simulink library "robot"  (Simulink 7.4)
settings: Solver=ode45  StartTime=0.0  StopTime=10.0  RelTol=1e-3
libraries: AtomicLibrary x3, BusImpl x1
settings Model: Creator=andrey  LastModifiedBy=andrey

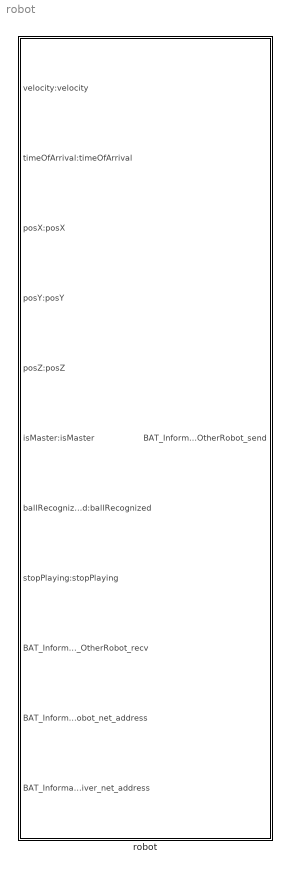
== system robot ==
  robot : Subsystem  Tag=id=_2CVEwKbHEeKVjd_905naCg

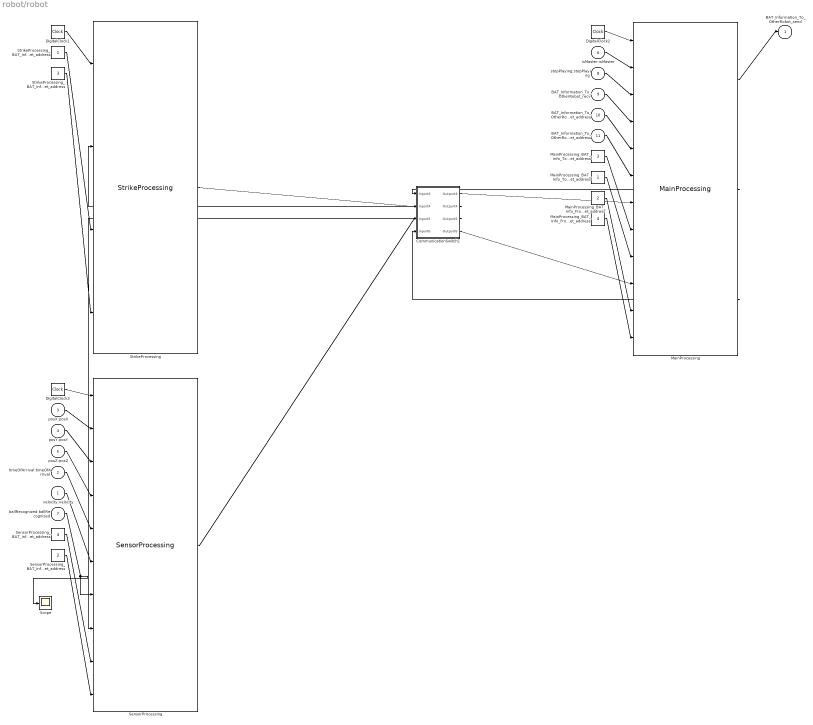
== system robot/robot ==
  velocity:velocity : Inport  Tag=id=_3IT1YKbHEeKVjd_905naCg  DataType=double  OutDataType=fixdt(1, 16)  OutScaling=2^0  OutDataTypeStr=double
  timeOfArrival:timeOfArrival : Inport  Tag=id=_3IliMKbHEeKVjd_905naCg  Port=2  DataType=double  OutDataType=fixdt(1, 16)  OutScaling=2^0  OutDataTypeStr=double
  posX:posX : Inport  Tag=id=_3I8HgKbHEeKVjd_905naCg  Port=3  DataType=double  OutDataType=fixdt(1, 16)  OutScaling=2^0  OutDataTypeStr=double
  posY:posY : Inport  Tag=id=_3JgvQKbHEeKVjd_905naCg  Port=4  DataType=double  OutDataType=fixdt(1, 16)  OutScaling=2^0  OutDataTypeStr=double
  posZ:posZ : Inport  Tag=id=_3KMEsKbHEeKVjd_905naCg  Port=5  DataType=double  OutDataType=fixdt(1, 16)  OutScaling=2^0  OutDataTypeStr=double
  isMaster:isMaster : Inport  Tag=id=_3Kp-wKbHEeKVjd_905naCg  Port=6  DataType=boolean  OutDataType=fixdt(1, 16)  OutScaling=2^0  OutDataTypeStr=boolean
  ballRecognized:ballRecognized : Inport  Tag=id=_3LJG8KbHEeKVjd_905naCg  Port=7  DataType=boolean  OutDataType=fixdt(1, 16)  OutScaling=2^0  OutDataTypeStr=boolean
  stopPlaying:stopPlaying : Inport  Tag=id=_3LnBAKbHEeKVjd_905naCg  Port=8  DataType=boolean  OutDataType=fixdt(1, 16)  OutScaling=2^0  OutDataTypeStr=boolean
  BAT_Information_To_OtherRobot_recv : Inport  Tag=id=_3MnGkKbHEeKVjd_905naCg  Port=9  UseBusObject=on  OutDataType=fixdt(1, 16)  OutScaling=2^0
      settings: BusObject=PacketBus
  BAT_Information_To_OtherRobot_net_address : Inport  Tag=id=_3MoUsKbHEeKVjd_905naCg  Port=10  DataType=uint8  OutDataType=fixdt(1, 16)  OutScaling=2^0  OutDataTypeStr=uint8
  BAT_Information_To_OtherRobot_receiver_net_address : Inport  Tag=id=_3MoUsabHEeKVjd_905naCg  Port=11  DataType=uint8  OutDataType=fixdt(1, 16)  OutScaling=2^0  OutDataTypeStr=uint8
  CommunicationSwitch1 : Subsystem  Tag=id=_2CVr0KbHEeKVjd_905naCg  LoadFcn=MainBusGenerator
  DigitalClock1 : DigitalClock  Tag=id=_2EqnEKbHEeKVjd_905naCg  SampleTime=0.0010
  DigitalClock2 : DigitalClock  Tag=id=_2ExUwKbHEeKVjd_905naCg  SampleTime=0.0010
  DigitalClock3 : DigitalClock  Tag=id=_2E1mMKbHEeKVjd_905naCg  SampleTime=0.0010
  MainProcessing : AtomicLibrary/MainProcessing  Tag=id=_2EwtsKbHEeKVjd_905naCg  SystemSampleTime=-1
  MainProcessing_BAT_Info_From_SensorProcessing1_net_address : Constant  Tag=id=_3Dm7kKbHEeKVjd_905naCg  Value=2  OutDataTypeMode=uint8  OutDataTypeStr=uint8
  MainProcessing_BAT_Info_From_SensorProcessing1_receiver_net_address : Constant  Tag=id=_4yrFcabHEeKVjd_905naCg  Value=4  OutDataTypeMode=uint8  OutDataTypeStr=uint8
  MainProcessing_BAT_Info_ToStrikeProcessing1_net_address : Constant  Tag=id=_3DVOwKbHEeKVjd_905naCg  Value=3  OutDataTypeMode=uint8  OutDataTypeStr=uint8
  MainProcessing_BAT_Info_ToStrikeProcessing1_receiver_net_address : Constant  Tag=id=_4ygtZabHEeKVjd_905naCg  OutDataTypeMode=uint8  OutDataTypeStr=uint8
  Scope : Scope
  SensorProcessing : AtomicLibrary/SensorProcessing  Tag=id=_2E0_IKbHEeKVjd_905naCg  SystemSampleTime=-1
  SensorProcessing_BAT_Info1_net_address : Constant  Tag=id=_3D-H8KbHEeKVjd_905naCg  Value=4  OutDataTypeMode=uint8  OutDataTypeStr=uint8
  SensorProcessing_BAT_Info1_receiver_net_address : Constant  Tag=id=_4yqeYabHEeKVjd_905naCg  Value=2  OutDataTypeMode=uint8  OutDataTypeStr=uint8
  StrikeProcessing : AtomicLibrary/StrikeProcessing  Tag=id=_2DLZUKbHEeKVjd_905naCg  SystemSampleTime=-1
  StrikeProcessing_BAT_Info1_net_address : Constant  Tag=id=_3DEJAKbHEeKVjd_905naCg  OutDataTypeMode=uint8  OutDataTypeStr=uint8
  StrikeProcessing_BAT_Info1_receiver_net_address : Constant  Tag=id=_4yh7gabHEeKVjd_905naCg  Value=3  OutDataTypeMode=uint8  OutDataTypeStr=uint8
  BAT_Information_To_OtherRobot_send : Outport  Tag=id=_3MntoKbHEeKVjd_905naCg  UseBusObject=on  OutDataType=fixdt(1, 16)  OutScaling=2^0
      settings: BusObject=PacketBus
  wires:
  DigitalClock1/1 -> StrikeProcessing/1
  DigitalClock2/1 -> MainProcessing/1
  DigitalClock3/1 -> SensorProcessing/1
  StrikeProcessing_BAT_Info1_net_address/1 -> StrikeProcessing/3
  MainProcessing_BAT_Info_ToStrikeProcessing1_net_address/1 -> MainProcessing/8
  MainProcessing_BAT_Info_From_SensorProcessing1_net_address/1 -> MainProcessing/11
  SensorProcessing_BAT_Info1_net_address/1 -> SensorProcessing/9
  MainProcessing/2 -> CommunicationSwitch1/1(Inport3)
  StrikeProcessing/1 -> CommunicationSwitch1/2(Inport4)
  CommunicationSwitch1/2(Outport4) -> StrikeProcessing/2
  CommunicationSwitch1/1(Outport3) -> MainProcessing/7
  MainProcessing_BAT_Info_ToStrikeProcessing1_receiver_net_address/1 -> MainProcessing/9
  StrikeProcessing_BAT_Info1_receiver_net_address/1 -> StrikeProcessing/4
  SensorProcessing/1 -> CommunicationSwitch1/3(Inport5)
  MainProcessing/3 -> CommunicationSwitch1/4(Inport6)
  CommunicationSwitch1/4(Outport6) -> MainProcessing/10
  CommunicationSwitch1/3(Outport5) -> SensorProcessing/8
  SensorProcessing_BAT_Info1_receiver_net_address/1 -> SensorProcessing/10
  MainProcessing_BAT_Info_From_SensorProcessing1_receiver_net_address/1 -> MainProcessing/12
  isMaster:isMaster/1 -> MainProcessing/2
  stopPlaying:stopPlaying/1 -> MainProcessing/3
  posY:posY/1 -> SensorProcessing/3
  velocity:velocity/1 -> SensorProcessing/6
  timeOfArrival:timeOfArrival/1 -> SensorProcessing/5
  posZ:posZ/1 -> SensorProcessing/4
  ballRecognized:ballRecognized/1 -> SensorProcessing/7, Scope/1
  posX:posX/1 -> SensorProcessing/2
  BAT_Information_To_OtherRobot_recv/1 -> MainProcessing/4
  MainProcessing/1 -> BAT_Information_To_OtherRobot_send/1
  BAT_Information_To_OtherRobot_receiver_net_address/1 -> MainProcessing/6
  BAT_Information_To_OtherRobot_net_address/1 -> MainProcessing/5

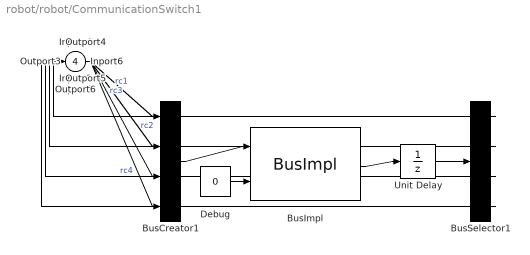
== system robot/robot/CommunicationSwitch1 ==
  Inport3 : Inport  Tag=id=_4yjJoKbHEeKVjd_905naCg  UseBusObject=on  OutDataType=fixdt(1, 16)  OutScaling=2^0
      settings: BusObject=PacketBus
  Inport4 : Inport  Tag=id=_4yjJoqbHEeKVjd_905naCg  Port=2  UseBusObject=on  OutDataType=fixdt(1, 16)  OutScaling=2^0
      settings: BusObject=PacketBus
  Inport5 : Inport  Tag=id=_4ysTkKbHEeKVjd_905naCg  Port=3  UseBusObject=on  OutDataType=fixdt(1, 16)  OutScaling=2^0
      settings: BusObject=PacketBus
  Inport6 : Inport  Tag=id=_4ysTkqbHEeKVjd_905naCg  Port=4  UseBusObject=on  OutDataType=fixdt(1, 16)  OutScaling=2^0
      settings: BusObject=PacketBus
  BusCreator1 : BusCreator  UseBusObject=on
      settings: BusObject=MainBus
  BusImpl : BusImpl/BusImpl
  BusSelector1 : BusSelector  OutputSignals=rc1,rc2,rc3,rc4
  Debug : Constant  Value=0  OutDataType=fixdt(1, 16)  OutScaling=2^0
  Unit Delay : UnitDelay  SampleTime=-1
  Outport3 : Outport  Tag=id=_4yjJoabHEeKVjd_905naCg  UseBusObject=on  OutDataType=fixdt(1, 16)  OutScaling=2^0
      settings: BusObject=PacketBus
  Outport4 : Outport  Tag=id=_4yjJo6bHEeKVjd_905naCg  Port=2  UseBusObject=on  OutDataType=fixdt(1, 16)  OutScaling=2^0
      settings: BusObject=PacketBus
  Outport5 : Outport  Tag=id=_4ysTkabHEeKVjd_905naCg  Port=3  UseBusObject=on  OutDataType=fixdt(1, 16)  OutScaling=2^0
      settings: BusObject=PacketBus
  Outport6 : Outport  Tag=id=_4ysTk6bHEeKVjd_905naCg  Port=4  UseBusObject=on  OutDataType=fixdt(1, 16)  OutScaling=2^0
      settings: BusObject=PacketBus
  wires:
  BusImpl/1 -> Unit Delay/1
  BusCreator1/1 -> BusImpl/1
  Unit Delay/1 -> BusSelector1/1
  Inport3/1 -> BusCreator1/1  "rc1"
  Inport4/1 -> BusCreator1/2  "rc2"
  Inport5/1 -> BusCreator1/3  "rc3"
  Inport6/1 -> BusCreator1/4  "rc4"
  BusSelector1/1 -> Outport3/1
  BusSelector1/2 -> Outport4/1
  BusSelector1/3 -> Outport5/1
  BusSelector1/4 -> Outport6/1
  Debug/1 -> BusImpl/2
